simulink model "sim_elicottero_2025"  (R2025b)
settings: Solver=VariableStepAuto  StopTime=100
values from neighbouring files (symbols this model uses):
  aero = evalin('base','aero')    [analisi_LQG.m]
  alpha_0 = deg2rad(10)    [dataset_elicottero.m]
  beta_0 = 0    [dataset_elicottero.m]
  Ddec_phys = [1.02312721492  -0.00983242196391; -0.0381188509726  0.136220944446]    [HINF_controllers.mat]    (also in Hinf_hinfstruct.m = Du *      Ddec_scaled *      Du_inv; Hinf_synthesis_full.m = Du *      Ddec_scaled *      inv(Du))
  den_2nd = [1, 2*zeta*omega_n, omega_n^2]    [dataset_elicottero.m]
  denFalpha = [1 32.8586170768]    [HINF_controllers.mat]
  denFbeta = [1 29.8807769231]    [HINF_controllers.mat]
  F1_0 = u0_nom(1)    [dataset_elicottero.m]
  F2_0 = u0_nom(2)    [dataset_elicottero.m]
  HalphaBeta = (C_angle_meas.'*Vinv*C_angle_meas) \      (C_angle_meas.'*Vinv)    [dataset_elicottero.m]
  K_hinfsyn = minreal(          Du *          K_hinfsyn_scaled *          Dy_inv,          1e-7)    [Hinf_hinfstruct.m]    (also in Hinf_synthesis_full.m = minreal(          Du *          K_hinfsyn_scaled *          )
  K_lqg_2dof = ss(      Ac_ctrl,      Bc_ctrl,      Cc_ctrl,      Dc_ctrl)    [LQG_reg_2DOF.m]
  K_lqg_int = ss(      Ac_ctrl,      [Bcr Bcy],      Cc_ctrl,      Dc_ctrl)    [LQG_con_integratore.m]
  K_mix = minreal(          Du *          K_mix_scaled *          Dy_inv,          1e-7)    [Hinf_hinfstruct.m]    (also in Hinf_synthesis_full.m = minreal(          Du *          K_mix_scaled *          Dy_i)
  K_mu = Du * K_mu_scaled * Dy_inv    [mu_synthesis.m]
  Kalpha_tuned = pid(          alphaScaledToPhys *          Kalpha_tuned_scaled.Kp,          alphaScaledToPhys *          Kalpha_tuned_scaled.Ki,          alphaScaledToPhys *          Kalpha_tuned_scaled.Kd,          Kalpha_tuned_scaled.Tf)    [Hinf_hinfstruct.m]    (also in Hinf_synthesis_full.m = pid(          alphaScaledToPhys * Kalpha_tuned_scaled.Kp,   )
  Kbeta_tuned = pid(          betaScaledToPhys *          Kbeta_tuned_scaled.Kp,          betaScaledToPhys *          Kbeta_tuned_scaled.Ki,          betaScaledToPhys *          Kbeta_tuned_scaled.Kd,          Kbeta_tuned_scaled.Tf)    [Hinf_hinfstruct.m]    (also in Hinf_synthesis_full.m = pid(          betaScaledToPhys * Kbeta_tuned_scaled.Kp,     )
  mx_eq = cos(alpha_0) * cos(beta_0)    [dataset_elicottero.m]
  my_eq = -sin(beta_0)    [dataset_elicottero.m]
  num_2nd = omega_n^2    (= 900)    [dataset_elicottero.m]
  numFalpha = [1.68743164033 27.5828822804]    [HINF_controllers.mat]
  numFbeta = [3.03350145907 0.0856653741444]    [HINF_controllers.mat]
  P_nom_ext = ss(      A_nom,      B_ext_nom,      Cy,      zeros(3,4))    [dataset_elicottero.m]
  tau_d_nom = 0.02    [dataset_elicottero.m]
  y_acc_eq = -p.g * sin(alpha_0)    [dataset_elicottero.m]
undefined symbols (not defined in the file or in its folder): act, sensor
libraries: simulink x21, slpidlib x4, cstblocks x2
(part 3 of 3)

== matlab function sim_elicottero_2025/Verifica Dinamica/Elicottero Dynamics ==
  data: x input; u input; x_dot output; p parameter
function x_dot = elicottero_dynamics(x, u, p)
    % ESTRAZIONE STATI
    alpha = x(1);
    alpha_dot = x(2);
    beta = x(3);
    beta_dot = x(4);
    
    % ESTRAZIONE INGRESSI

    F1 = u(1);
    F2 = u(2);

                 
    % 1. Vettore velocità angolare nel sistema Body (omega_B)
    % Il Pitch (alpha_dot) ruota attorno all'asse Y_body.
    % Lo Yaw (beta_dot) ruota attorno all'asse Z_inerziale, che proiettato in Body diventa [-sin(alpha); 0; cos(alpha)]
    omega_body = [-beta_dot * sin(alpha); 
                   alpha_dot; 
                   beta_dot * cos(alpha)];
                   
    % 2. Vettore posizione del centro aerodinamico (i rotori a distanza l sull'asse X_body)
    r_cp = [p.l; 0; 0];
    
    % 3. Velocità lineare del corpo dovuta alla rotazione (v = omega x r)
    v_corpo_body = cross(omega_body, r_cp); 
    % (Il risultato analitico sarà: [0; p.l * beta_dot * cos(alpha); -p.l * alpha_dot])
    
    
    % 5. VELOCITÀ RELATIVA VERA (Vento esterno - Velocità del corpo)
    v_rel_body  = - v_corpo_body; 
    v_rel_norm  = norm(v_rel_body);
    
    % Calcolo Forze Aerodinamiche
    % NOTA: Per pulizia del codice, in futuro potresti spostare rho e Cd_A 
    % all'interno della struct dei parametri 'p'
    rho = 1.225; % Densità dell'aria [kg/m^3]
    Cd_A = [0.5; 0.6; 1.2]; % Prodotto Cd * Area per gli assi [X; Y; Z]
    % Bracci da $0.25$ e $0.30$ m: Sono lunghezze tipiche dei bracci di un 
    % elicottero didattico da laboratorio a 2 gradi di libertà, come i 
    % classici modelli Quanser Aero o i TRMS (Twin Rotor MIMO System)
    
    F_drag_body = 0.5 * rho * Cd_A .* v_rel_body * v_rel_norm;
    
    % Calcolo Coppie di Disturbo
    % Assumiamo che la forza aerodinamica agisca con braccio pari a p.l
    tau_wind_alpha = -F_drag_body(3) * p.l; % Forza verticale genera coppia di pitch
    tau_wind_beta  = F_drag_body(2) * p.l; % Forza laterale genera coppia di yaw
    
    % DINAMICA: Inerzia variabile di yaw
    J_beta = p.J_y * sin(alpha)^2 + (p.J_z + p.m*p.l^2)*cos(alpha)^2 + p.I_b;
    
    % EQUAZIONI DEL MOTO (Accelerazioni)
    alpha_ddot = (-p.c_alpha*alpha_dot ...
                  - p.m*p.g*p.l*sin(alpha) ...
                  + p.l*F1*cos(beta) ...
                  + p.eps_p*p.l*F2*sin(beta) ...
                  ) / p.J_alpha;

    beta_ddot = (-p.c_beta*beta_dot ...
                 + p.l*F2*cos(alpha) ...
                 + p.eps_y*p.l*F1*sin(alpha) ...
                 ) / J_beta;
    % USCITA: Vettore colonna delle derivate dello stato
    x_dot = [alpha_dot; alpha_ddot; beta_dot; beta_ddot];
end

== matlab function sim_elicottero_2025/Hinf_nl/Elicottero Dynamics1 ==
  data: x input; u input; x_dot output; p parameter
function x_dot = elicottero_dynamics(x, u, p)
    % ESTRAZIONE STATI
    alpha = x(1);
    alpha_dot = x(2);
    beta = x(3);
    beta_dot = x(4);
    
    % ESTRAZIONE INGRESSI

    F1 = u(1);
    F2 = u(2);

    d_alpha = u(3);
    d_beta  = u(4);
                 
    % 1. Vettore velocità angolare nel sistema Body (omega_B)
    % Il Pitch (alpha_dot) ruota attorno all'asse Y_body.
    % Lo Yaw (beta_dot) ruota attorno all'asse Z_inerziale, che proiettato in Body diventa [-sin(alpha); 0; cos(alpha)]
    omega_body = [-beta_dot * sin(alpha); 
                   alpha_dot; 
                   beta_dot * cos(alpha)];
                   
    % 2. Vettore posizione del centro aerodinamico (i rotori a distanza l sull'asse X_body)
    r_cp = [p.l; 0; 0];
    
    % 3. Velocità lineare del corpo dovuta alla rotazione (v = omega x r)
    v_corpo_body = cross(omega_body, r_cp); 
    % (Il risultato analitico sarà: [0; p.l * beta_dot * cos(alpha); -p.l * alpha_dot])
    
    
    % 5. VELOCITÀ RELATIVA VERA (Vento esterno - Velocità del corpo)
    v_rel_body  = - v_corpo_body; 
    v_rel_norm  = norm(v_rel_body);
    
    % Calcolo Forze Aerodinamiche
    % NOTA: Per pulizia del codice, in futuro potresti spostare rho e Cd_A 
    % all'interno della struct dei parametri 'p'
    rho = 1.225; % Densità dell'aria [kg/m^3]
    Cd_A = [0.5; 0.6; 1.2]; % Prodotto Cd * Area per gli assi [X; Y; Z]
    % Bracci da $0.25$ e $0.30$ m: Sono lunghezze tipiche dei bracci di un 
    % elicottero didattico da laboratorio a 2 gradi di libertà, come i 
    % classici modelli Quanser Aero o i TRMS (Twin Rotor MIMO System)
    
    F_drag_body = 0.5 * rho * Cd_A .* v_rel_body * v_rel_norm;
    
    % Calcolo Coppie di Disturbo
    % Assumiamo che la forza aerodinamica agisca con braccio pari a p.l
    tau_wind_alpha = -F_drag_body(3) * p.l; % Forza verticale genera coppia di pitch
    tau_wind_beta  = F_drag_body(2) * p.l; % Forza laterale genera coppia di yaw
    
    % DINAMICA: Inerzia variabile di yaw
    J_beta = p.J_y * sin(alpha)^2 + (p.J_z + p.m*p.l^2)*cos(alpha)^2 + p.I_b;
    
    % EQUAZIONI DEL MOTO (Accelerazioni)
    alpha_ddot = (-p.c_alpha*alpha_dot ...
                  - p.m*p.g*p.l*sin(alpha) ...
                  + p.l*F1*cos(beta) ...
                  + p.eps_p*p.l*F2*sin(beta) ...
                  + d_alpha) / p.J_alpha;

    beta_ddot = (-p.c_beta*beta_dot ...
                 + p.l*F2*cos(alpha) ...
                 + p.eps_y*p.l*F1*sin(alpha) ...
                 + d_beta) / J_beta;
    % USCITA: Vettore colonna delle derivate dello stato
    x_dot = [alpha_dot; alpha_ddot; beta_dot; beta_ddot];
end

== matlab function sim_elicottero_2025/mu_controller_nl/Elicottero Dynamics ==
  data: x input; u input; x_dot output; p parameter
function x_dot = elicottero_dynamics(x, u, p)
    % ESTRAZIONE STATI
    alpha = x(1);
    alpha_dot = x(2);
    beta = x(3);
    beta_dot = x(4);
    
    % ESTRAZIONE INGRESSI

    F1 = u(1);
    F2 = u(2);

    d_alpha = u(3);
    d_beta  = u(4);
                 
    % 1. Vettore velocità angolare nel sistema Body (omega_B)
    % Il Pitch (alpha_dot) ruota attorno all'asse Y_body.
    % Lo Yaw (beta_dot) ruota attorno all'asse Z_inerziale, che proiettato in Body diventa [-sin(alpha); 0; cos(alpha)]
    omega_body = [-beta_dot * sin(alpha); 
                   alpha_dot; 
                   beta_dot * cos(alpha)];
                   
    % 2. Vettore posizione del centro aerodinamico (i rotori a distanza l sull'asse X_body)
    r_cp = [p.l; 0; 0];
    
    % 3. Velocità lineare del corpo dovuta alla rotazione (v = omega x r)
    v_corpo_body = cross(omega_body, r_cp); 
    % (Il risultato analitico sarà: [0; p.l * beta_dot * cos(alpha); -p.l * alpha_dot])
    
    
    % 5. VELOCITÀ RELATIVA VERA (Vento esterno - Velocità del corpo)
    v_rel_body  = - v_corpo_body; 
    v_rel_norm  = norm(v_rel_body);
    
    % Calcolo Forze Aerodinamiche
    % NOTA: Per pulizia del codice, in futuro potresti spostare rho e Cd_A 
    % all'interno della struct dei parametri 'p'
    rho = 1.225; % Densità dell'aria [kg/m^3]
    Cd_A = [0.5; 0.6; 1.2]; % Prodotto Cd * Area per gli assi [X; Y; Z]
    % Bracci da $0.25$ e $0.30$ m: Sono lunghezze tipiche dei bracci di un 
    % elicottero didattico da laboratorio a 2 gradi di libertà, come i 
    % classici modelli Quanser Aero o i TRMS (Twin Rotor MIMO System)
    
    F_drag_body = 0.5 * rho * Cd_A .* v_rel_body * v_rel_norm;
    
    % Calcolo Coppie di Disturbo
    % Assumiamo che la forza aerodinamica agisca con braccio pari a p.l
    tau_wind_alpha = -F_drag_body(3) * p.l; % Forza verticale genera coppia di pitch
    tau_wind_beta  = F_drag_body(2) * p.l; % Forza laterale genera coppia di yaw
    
    % DINAMICA: Inerzia variabile di yaw
    J_beta = p.J_y * sin(alpha)^2 + (p.J_z + p.m*p.l^2)*cos(alpha)^2 + p.I_b;
    
    % EQUAZIONI DEL MOTO (Accelerazioni)
    alpha_ddot = (-p.c_alpha*alpha_dot ...
                  - p.m*p.g*p.l*sin(alpha) ...
                  + p.l*F1*cos(beta) ...
                  + p.eps_p*p.l*F2*sin(beta) ...
                  + d_alpha) / p.J_alpha;

    beta_ddot = (-p.c_beta*beta_dot ...
                 + p.l*F2*cos(alpha) ...
                 + p.eps_y*p.l*F1*sin(alpha) ...
                 + d_beta) / J_beta;
    % USCITA: Vettore colonna delle derivate dello stato
    x_dot = [alpha_dot; alpha_ddot; beta_dot; beta_ddot];
end

== matlab function sim_elicottero_2025/Hinf_nl/Sensori IMU1 ==
  data: x input; y_ideal output; p parameter
function y_ideal = sensori_imu(x, p)
    % ESTRAZIONE STATI RILEVANTI
    alpha = x(1);
    beta = x(3);
    
    % EQUAZIONI DEI SENSORI (Misure ideali a 3 uscite)
    y_acc = -p.g * sin(alpha);
    mx = cos(alpha) * cos(beta);
    my = -sin(beta);
    
    % USCITA: Vettore colonna 3x1
    y_ideal = [y_acc; mx; my];
end
